simulink model "LSMCPWM_9lvl"  (R2018a)
settings: Solver=VariableStepAuto  StartTime=0.0  StopTime=0.1  FixedStep=0.1/1000  RelTol=1e-3
libraries: powerlib x24, simulink x8
settings Model: Creator=Muhammad Osama  LastModifiedBy=Muhammad Osama

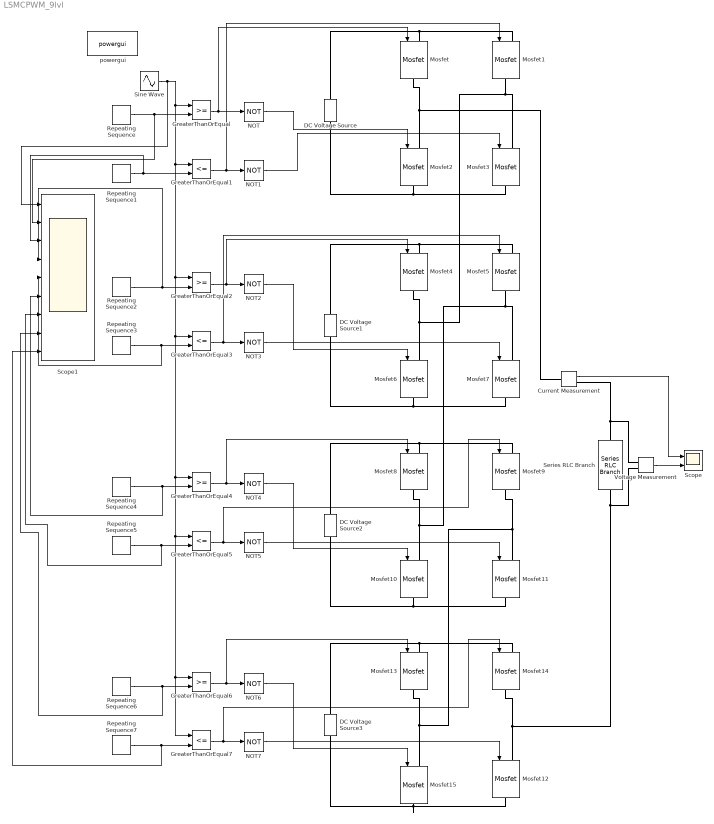
== system LSMCPWM_9lvl ==
  Current Measurement : powerlib/Measurements/Current Measurement  PhasorSimulation=off  OutputType=Complex  PSBequivalent=0
  DC Voltage Source{,1..3} (4 alike) : powerlib/Electrical Sources/DC Voltage Source  Amplitude=10  Measurements=None
  GreaterThanOrEqual{,2,4,6} (4 alike) : RelationalOperator  OutDataTypeStr=boolean  RndMeth=Simplest  InputSameDT=on
  GreaterThanOrEqual{1,3,5,7} (4 alike) : RelationalOperator  Operator=<=  OutDataTypeStr=boolean  RndMeth=Simplest  InputSameDT=on
  Mosfet{,1..15} (16 alike) : powerlib/Power Electronics/Mosfet  Ron=0.1  Lon=0  Rd=0.01  Vfd=0  IC=0  Rs=1e5  Cs=inf  Measurements=off
  NOT{,1..7} (8 alike) : Logic  Operator=NOT  IconShape=distinctive  OutDataTypeStr=boolean
  Repeating Sequence : simulink/Sources/Repeating Sequence  rep_seq_t=[0 0.5 1]/1000  rep_seq_y=[0.75 1 0.75]
  Repeating Sequence1 : simulink/Sources/Repeating Sequence  rep_seq_t=[0 0.5 1]/1000  rep_seq_y=[0.5 0.75 0.5]
  Repeating Sequence2 : simulink/Sources/Repeating Sequence  rep_seq_t=[0 0.5 1]/1000  rep_seq_y=[0.25 0.5 0.25]
  Repeating Sequence3 : simulink/Sources/Repeating Sequence  rep_seq_t=[0 0.5 1]/1000  rep_seq_y=[0 0.25 0]
  Repeating Sequence4 : simulink/Sources/Repeating Sequence  rep_seq_t=[0 0.5 1]/1000  rep_seq_y=[-0.25 0 -0.25]
  Repeating Sequence5 : simulink/Sources/Repeating Sequence  rep_seq_t=[0 0.5 1]/1000  rep_seq_y=[-0.5 -0.25 -0.5]
  Repeating Sequence6 : simulink/Sources/Repeating Sequence  rep_seq_t=[0 0.5 1]/1000  rep_seq_y=[-0.75 -0.5 -0.75]
  Repeating Sequence7 : simulink/Sources/Repeating Sequence  rep_seq_t=[0 0.5 1]/1000  rep_seq_y=[-1 -0.75 -1]
  Scope : Scope  NumInputPorts=2
  Scope1 : Scope  NumInputPorts=9
  Series RLC Branch : powerlib/Elements/Series RLC Branch  LConnTagsString=__new0  RConnTagsString=__new0  BranchType=R  Resistance=10  Inductance=400e-6  SetiL0=off  InitialCurrent=0  Capacitance=3e-6  Setx0=off  InitialVoltage=0  Measurements=None
  Sine Wave : Sin  Frequency=2*pi*50  SampleTime=0
  Voltage Measurement : powerlib/Measurements/Voltage Measurement  PhasorSimulation=off  OutputType=Complex  PSBequivalent=0
  powergui : powerlib/powergui  Priority=1  SimulationMode=Discrete  SampleTime=50e-6  frequency=60  Iterations=50  frequencyindice=0  Pbase=100e6  ErrMax=1e-4  UnitsV=kV  UnitsW=MW  buscounter=0  FunctionMessages=off  echomessages=off  EnableUseOfTLC=off  CurrentSourceSwitches=off  DisableSnubberDevices=off  DisableRonSwitches=off  DisableVfSwitches=off  DisplayEquations=off  SolverType=Tustin/Backward Euler (TBE)  Interpol=off  ExternalGateDelay=off  methode=off  Ts=100  x0status=blocks  SPID=off  SwTol=0  HookPort=off  RestoreLinks=warning  ResistiveCurrentMeasurement=off  Frange=[0:2:500]  Ylog=off  Xlog=on  ShowGrid=off  save=off  variable=ZData  structure=0  ZoomFFT=off  StartTime=0.0  cycles=1  DisplayStyle=1  fundamental=60  FreqAxis=off  MaxFrequency=1000  frequencyindicesteady=1  RmsSteady=1  display=off
  wires:
  GreaterThanOrEqual/1 -> Mosfet/1, NOT/1
  GreaterThanOrEqual1/1 -> Mosfet1/1, NOT1/1
  GreaterThanOrEqual2/1 -> Mosfet4/1, NOT2/1
  GreaterThanOrEqual3/1 -> Mosfet5/1, NOT3/1
  NOT1/1 -> Mosfet3/1
  NOT/1 -> Mosfet2/1
  NOT3/1 -> Mosfet7/1
  NOT2/1 -> Mosfet6/1
  Voltage Measurement/1 -> Scope/2
  Current Measurement/1 -> Scope/1
  Repeating Sequence/1 -> Scope1/2, GreaterThanOrEqual/2
  Repeating Sequence1/1 -> Scope1/3, GreaterThanOrEqual1/2
  Repeating Sequence2/1 -> Scope1/4, GreaterThanOrEqual2/2
  Repeating Sequence3/1 -> Scope1/5, GreaterThanOrEqual3/2
  Repeating Sequence4/1 -> Scope1/6, GreaterThanOrEqual4/2
  Repeating Sequence5/1 -> Scope1/7, GreaterThanOrEqual5/2
  NOT5/1 -> Mosfet11/1
  NOT4/1 -> Mosfet10/1
  GreaterThanOrEqual4/1 -> Mosfet8/1, NOT4/1
  GreaterThanOrEqual5/1 -> Mosfet9/1, NOT5/1
  Repeating Sequence6/1 -> Scope1/8, GreaterThanOrEqual6/2
  GreaterThanOrEqual7/1 -> Mosfet14/1, NOT7/1
  GreaterThanOrEqual6/1 -> Mosfet13/1, NOT6/1
  Sine Wave/1 -> Scope1/1, GreaterThanOrEqual4/1, GreaterThanOrEqual6/1, GreaterThanOrEqual7/1, GreaterThanOrEqual5/1, GreaterThanOrEqual3/1, GreaterThanOrEqual2/1, GreaterThanOrEqual1/1, GreaterThanOrEqual/1
  NOT7/1 -> Mosfet12/1
  NOT6/1 -> Mosfet15/1
  Repeating Sequence7/1 -> Scope1/9, GreaterThanOrEqual7/2
  connections:
  Mosfet/LConn1 -- DC Voltage Source/RConn1 -- Mosfet1/LConn1
  Mosfet/RConn1 -- Current Measurement/LConn1 -- Mosfet2/LConn1
  Mosfet3/RConn1 -- DC Voltage Source/LConn1 -- Mosfet2/RConn1
  Mosfet4/LConn1 -- DC Voltage Source1/RConn1 -- Mosfet5/LConn1
  Mosfet4/RConn1 -- Mosfet3/LConn1 -- Mosfet1/RConn1 -- Mosfet6/LConn1
  Mosfet6/RConn1 -- DC Voltage Source1/LConn1 -- Mosfet7/RConn1
  Series RLC Branch/LConn1 -- Voltage Measurement/LConn1 -- Current Measurement/RConn1
  Mosfet11/RConn1 -- Mosfet10/RConn1 -- DC Voltage Source2/LConn1
  Mosfet8/RConn1 -- Mosfet7/LConn1 -- Mosfet5/RConn1 -- Mosfet10/LConn1
  Mosfet9/LConn1 -- Mosfet8/LConn1 -- DC Voltage Source2/RConn1
  Mosfet14/RConn1 -- Voltage Measurement/LConn2 -- Series RLC Branch/RConn1 -- Mosfet12/LConn1
  DC Voltage Source3/RConn1 -- Mosfet14/LConn1 -- Mosfet13/LConn1
  DC Voltage Source3/LConn1 -- Mosfet15/RConn1 -- Mosfet12/RConn1
  Mosfet13/RConn1 -- Mosfet15/LConn1 -- Mosfet11/LConn1 -- Mosfet9/RConn1
